simulink model "hil_sil_plant"  (R2022b)
settings: Solver=FixedStepAuto  StartTime=0.0  StopTime=inf  FixedStep=0.001  RelTol=1e-3
undefined symbols (not defined in the file): Ended, ind, Single
libraries: canmsglib x8, speedgoatlib_IO614 x5, speedgoatlib_IO191 x5, slrealtimeiplib x3, AMK_comms_plant_lib x1, BMS_plant_lib x1, slrealtimeutilitieslib x1, etargetslib x1
settings Model: Creator=LinF  LastModifiedBy=maxfa
settings SolverCC: ConcurrentTasks=on  PositivePriorityOrder=on
settings OptimizationCC: BlockReduction=off  OptimizeBlockIOStorage=off
settings DebuggingCC: TasksWithSamePriorityMsg=none
settings HardwareCC: ProdBitPerLong=64  ProdLongLongMode=on  ProdHWDeviceType=Intel->x86-64 (Linux 64)
settings RTWCC: Description=Simulink Real-Time  SystemTargetFile=slrealtime.tlc  TemplateMakefile=slrealtime_default_tmf  Toolchain=Simulink Real-Time Toolchain  BuildConfiguration=Faster Runs  CodeExecutionProfiling=on  TargetLang=C++

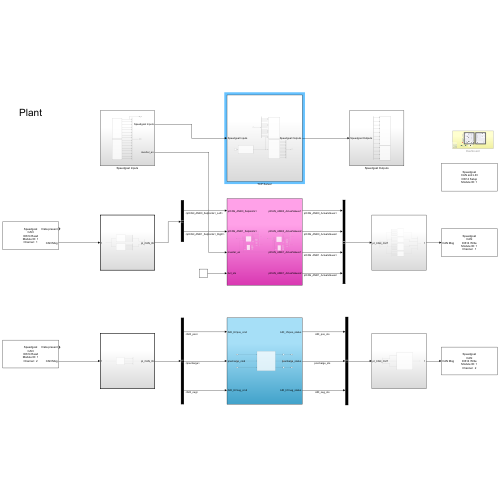
[thumbnail: Simulink's stored preview of the top-level diagram]
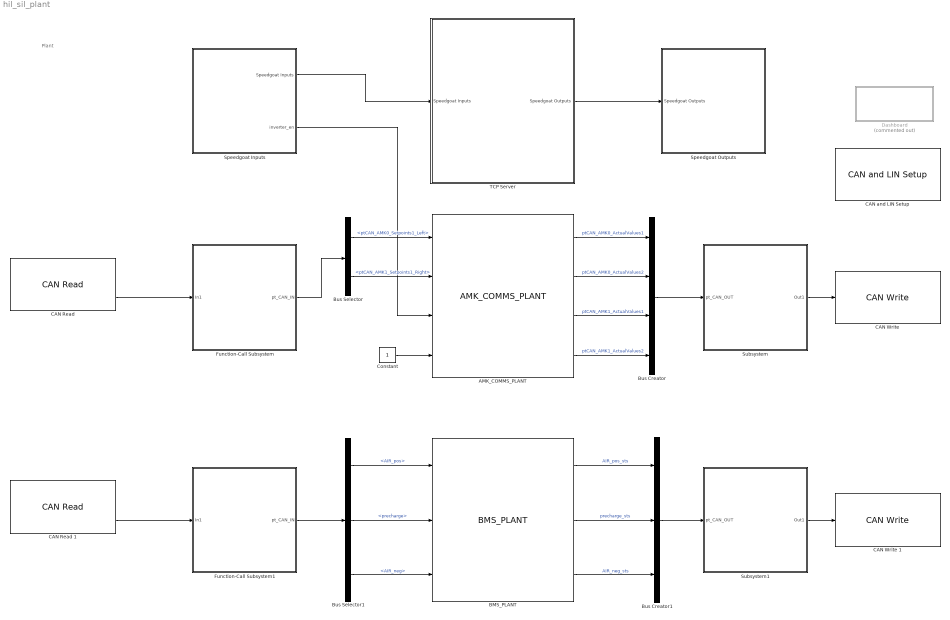
== system hil_sil_plant ==
  note: Plant
  AMK_COMMS_PLANT : AMK_comms_plant_lib/AMK_COMMS_PLANT  SystemSampleTime=-1  VariantActivationTime=update diagram  Latency=0  AutoFrameSizeCalculation=off
  BMS_PLANT : BMS_plant_lib/BMS_PLANT  SystemSampleTime=-1  VariantActivationTime=update diagram  Latency=0  AutoFrameSizeCalculation=off
  Bus Creator : BusCreator  Inputs=4
  Bus Creator1 : BusCreator  Inputs=3
  Bus Selector : BusSelector  OutputSignals=ptCAN_AMK0_Setpoints1_Left,ptCAN_AMK1_Setpoints1_Right
  Bus Selector1 : BusSelector  OutputSignals=AIR_pos,precharge,AIR_neg
  "CAN Read " : speedgoatlib_IO614/CAN Read   moduleType=IO614  id=1  channel=1  canType=CAN (HS)  useBusOut=off  HasMulRead=Single Read from Buffer (FIFO)  MsgIDlist=[1 2]  isEFF=off  LabelInHex=on  enableInput=off  ts=-1  initValues=[614 1 -1 0 1 1 0 0 0 1 2 1 2]
      settings: SourceProductName=Simulink Real-Time: Speedgoat I/O Blockset
  CAN Read 1 : speedgoatlib_IO614/CAN Read   moduleType=IO614  id=1  channel=2  canType=CAN (HS)  useBusOut=off  HasMulRead=Single Read from Buffer (FIFO)  MsgIDlist=[1 2]  isEFF=off  LabelInHex=on  enableInput=off  ts=-1  initValues=[614 1 -1 1 1 1 0 0 0 1 2 1 2]
      settings: SourceProductName=Simulink Real-Time: Speedgoat I/O Blockset
  "CAN Write " : speedgoatlib_IO614/CAN Write   moduleType=IO614  id=1  channel=1  canType=CAN (HS)  useBusIn=off  numOfMsg=4  enableInput=off  enableStatusPort=off  initValues=[614 1 0.01 0 1 1 0 4 0 0]  ts=0.01
      settings: SourceProductName=Simulink Real-Time: Speedgoat I/O Blockset
  CAN Write 1 : speedgoatlib_IO614/CAN Write   moduleType=IO614  id=1  channel=2  canType=CAN (HS)  useBusIn=off  numOfMsg=1  enableInput=off  enableStatusPort=off  initValues=[614 1 0.008 1 1 1 0 1 0 0]  ts=0.008
      settings: SourceProductName=Simulink Real-Time: Speedgoat I/O Blockset
  "CAN and LIN Setup " : speedgoatlib_IO614/CAN and LIN Setup   moduleInitValues="[614    1    1   -1   -1]"  id=1  moduleType=IO614  pciSlot=-1  canChn1=CAN (HS)  canChn2=CAN (HS)  canChn3=Disabled  canChn4=Disabled  linChn1=Disabled  linChn2=Disabled  canInitStructArray=[]  canTermStructArray=[]  canChn1InitValues="[2   4   1  31   8   2   1   5   2]"  arbBdrChn1=500 kBaud  arbManBdrChn1=[4,1,31,8]  fdBdrChn1=5.0 MBaud  fdManBdrChn1=[2,1,5,2]  canChn2InitValues="[2   4   1  31   8   2   1   5   2]"  arbBdrChn2=500 kBaud  arbManBdrChn2=[4,1,31,8]  fdBdrChn2=5.0 MBaud  fdManBdrChn2=[2,1,5,2]  canChn3InitValues="[1   2   1  31   8   2   1   5   2]"  arbBdrChn3=1.0 MBaud  arbManBdrChn3=[2,1,31,8]  fdBdrChn3=5.0 MBaud  fdManBdrChn3=[2,1,5,2]  canChn4InitValues="[1   2   1  31   8   2   1   5   2]"  arbBdrChn4=1.0 MBaud  arbManBdrChn4=[2,1,31,8]  fdBdrChn4=5.0 MBaud  fdManBdrChn4=[2,1,5,2]  bdrLIN1=19200  linChn1InitValues="[1  19200]"  bdrLIN2=19200  linChn2InitValues="[1  19200]"
      settings: LibrarySourceBlock=speedgoatlib_CANLIN_OfA2/CAN and LIN Setup
  Constant : Constant
  Dashboard : Subsystem  Commented=on
  Function-Call Subsystem : Subsystem  TreatAsAtomicUnit=on
  Function-Call Subsystem1 : Subsystem  TreatAsAtomicUnit=on
  Speedgoat Inputs : Subsystem
  Speedgoat Outputs : Subsystem
  Subsystem : Subsystem
  Subsystem1 : Subsystem
  TCP Server : Subsystem
  wires:
  Subsystem/1(Out1) -> "CAN Write "/1
  Function-Call Subsystem/1(pt_CAN_IN) -> Bus Selector/1
  Bus Selector/2 -> AMK_COMMS_PLANT/2  "<ptCAN_AMK1_Setpoints1_Right>"
  Bus Selector/1 -> AMK_COMMS_PLANT/1  "<ptCAN_AMK0_Setpoints1_Left>"
  Speedgoat Inputs/2(inverter_en) -> AMK_COMMS_PLANT/3
  AMK_COMMS_PLANT/1 -> Bus Creator/1  "ptCAN_AMK0_ActualValues1"
  AMK_COMMS_PLANT/2 -> Bus Creator/2  "ptCAN_AMK0_ActualValues2"
  AMK_COMMS_PLANT/3 -> Bus Creator/3  "ptCAN_AMK1_ActualValues1"
  AMK_COMMS_PLANT/4 -> Bus Creator/4  "ptCAN_AMK1_ActualValues2"
  Bus Creator/1 -> Subsystem/1(pt_CAN_OUT)
  Function-Call Subsystem1/1(pt_CAN_IN) -> Bus Selector1/1
  Bus Selector1/1 -> BMS_PLANT/1  "<AIR_pos>"
  Bus Selector1/3 -> BMS_PLANT/3  "<AIR_neg>"
  Subsystem1/1(Out1) -> CAN Write 1/1
  BMS_PLANT/1 -> Bus Creator1/1  "AIR_pos_sts"
  BMS_PLANT/2 -> Bus Creator1/2  "precharge_sts"
  BMS_PLANT/3 -> Bus Creator1/3  "AIR_neg_sts"
  Bus Creator1/1 -> Subsystem1/1(pt_CAN_OUT)
  "CAN Read "/2 -> Function-Call Subsystem/1(In1)
  CAN Read 1/2 -> Function-Call Subsystem1/1(In1)
  Bus Selector1/2 -> BMS_PLANT/2  "<precharge>"
  Constant/1 -> AMK_COMMS_PLANT/4
  TCP Server/1(Speedgoat Outputs) -> Speedgoat Outputs/1(Speedgoat Outputs)
  Speedgoat Inputs/1(Speedgoat Inputs) -> TCP Server/1(Speedgoat Inputs)

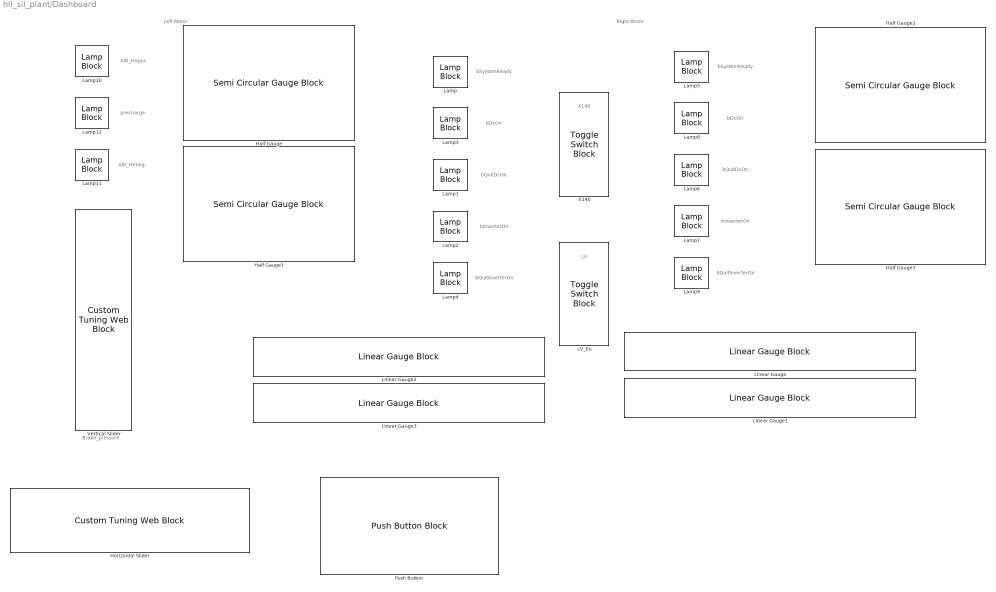
== system hil_sil_plant/Dashboard ==
  note: Brake_pressure
  note: LV
  note: X140
  note: Left Motor
  note: bQuitInverterOn
  note: bInverterOn
  note: bQuitDcOn
  note: bDcOn
  note: bSystemReady
  note: bDcOn
  note: bQuitDcOn
  note: bSystemReady
  note: bInverterOn
  note: bQuitInverterOn
  note: Right Motor
  note: AIR_HVpos
  note: precharge
  note: AIR_HVneg
  Half Gauge : SemiCircularGaugeBlock  LabelPosition=Bottom  ScaleMax=20000  TickInterval=2000
  Half Gauge1 : SemiCircularGaugeBlock  LabelPosition=Bottom  ScaleMax=1000  TickInterval=100
  Half Gauge2 : SemiCircularGaugeBlock  LabelPosition=Bottom  ScaleMax=20000  TickInterval=2000
  Half Gauge3 : SemiCircularGaugeBlock  LabelPosition=Bottom  ScaleMax=1000  TickInterval=100
  Horizontal Slider : CustomTuningWebBlock  LabelPosition=Hide  ShowInitialText=on  Configuration="{\"components\":[{\"name\":\"LinearScaleComponent\",\"settings\":{\"bounds\":{\"max\":4095,\"min\":0,\"tickInterval\":\"auto\"},\"internalTickHeightScaleFactor\":0.5,\"labelColor\":[255,255,200],\"labelFont\":{\"font\":\"Arial\",\"fontSize\":12},\"labelOffset\":0.05,\"labelTransparency\":1,\"needleImage\":{\"size\":[596,842],\"src\":\"data:image\\/svg+xml;base64,PD94bWwgdmVyc2lvbj0iMS4wIiBlbmNvZGluZz0idXRmLTgiPz4NCjwhLS0gR2VuZXJhdG9yOiBBZG9iZSBJbGx1c3RyYXRvciAyNS4wLjAsIFNWRyBFeHBvcnQgUGx1Zy1JbiAuIFNWRyBWZXJzaW9uOiA2LjAwIEJ1aWxkIDApICAtLT4NCjxzdmcgdmVyc2lvbj0iMS4xIg0KCSBpZD0ic3ZnOCIgeG1sbnM6Y2M9Imh0dHA6Ly9jcmVhdGl2ZWNvbW1vbnMub3JnL25zIyIgeG1sbnM6ZGM9Imh0dHA6Ly9wdXJsLm9yZy9kYy9lbGVtZW50cy8xLjEvIiB4bWxuczppbmtzY2FwZT0iaHR0cDovL3d3dy5pbmtzY2FwZS5vcmcvbmFtZXNw ...(+2420 chars)\",\"srcOrientation\":\"Right\"},\"needleOffset\":[-0.8044596912521441,-0.0642123287671233],\"needleSize\":{\"height\":0.4337797619047619,\"width\":0.07668067226890757},\"position\":[0.2829861111111111,0.04398634453781513,0.9196428571428571,0.6088789682539683],\"referencePoint\":\"auto\",\"scaleColors\":[],\"scaleColorsSize\":0.2,\"scaleDirection\":\"LR\",\"showLabels\":1,\"showMinorTicks\":0,\"showSpanLine\":1,\"showTicks\":1,\"tickColor\":[252,252,197],\"tickTransparency\":1,\"valueBarColor\":[0,114,189],\"valueBarOffset\":-0.27,\"valueBarSize\":0.1,\"valueBarTransparency\":1}},{\"name\":\"BackgroundImageComponent\",\"settings\":{\"image\":{\"size\":[380,101],\"src\":\"data:image\\/svg+xml;base64,PHN2ZyB4bWxucz0iaHR0cDovL3d3dy53My5vcmcvMjAwMC9zdmciIHhtbG5zOnhsaW5rPSJodHRwOi8vd3d3LnczLm9yZy8xOTk5L3hsaW5rIiB2aWV3Qm94PSIwIDAgMzgwIDEwMSI+PGRlZnM+PHN0eWxlPi5jbHMtMXtmaWxsOiMwMDJiNDI7fS5jbHMtMntmaWxsOiM0MjcwODI7fS5jbHMtM3tmaWxsOnVybCgjcmFkaWFsLWdyYWRpZW50KTt9LmNscy00e2ZpbGw6I2M4YzhjODtzdHJva2U6IzAwMDt9PC9zdHlsZT48cmFkaWFsR3JhZGllbnQgaWQ9InJhZGlhbC1ncmFkaWVudCIgY3g9IjE5MCIgY3k9IjUwLjUiIHI9IjI2OS4yMSIgZ3JhZGllbnRVbml0cz0idXNlclNwYWNlT25Vc2UiPjxzdG9wIG9mZnNldD0iMC4wMSIgc3RvcC1jb2xvcj0iIzNlNGY1OCIvPjxzdG9wIG9mZnNldD0iMC4wNiIgc3RvcC1jb2xvcj0iIzQ0NTc2MSIvPjxzdG9wIG9mZnNldD0iMC4xNSIgc3RvcC1jb2xvcj0iIzU1NmE3NiIvPjxzdG9wIG9mZnNldD0iMC4yNSIgc3RvcC1jb2xvcj0iIzZkODg5NSIvPjxzdG9wIG9mZnNldD0iMC4zOCIgc3RvcC1jb2xvcj0iIzhmYjJjMyIvPjxzdG9wIG9mZnNldD0iMC41MiIgc3RvcC1jb2xvcj0iI2I2ZTRmYSIvPjxzdG9wIG9mZnNldD0iMSIgc3RvcC1jb2xvcj0iIzE1NDY1NyIvPjwvcmFkaWFsR3JhZGllbnQ+PC9kZWZzPjxnIGlkPSJmcmFtZSI+PGcgaWQ9IkxheWVyXzIiIGRhdGEtbmFtZT0iTGF5ZXIgMiI+PGcgaWQ9IkxheWVyXzEtMiIgZGF0YS1uYW1lPSJMYXllciAxLTIiPjxyZWN0IGlkPSJyZWN0MTAzNiIgY2xhc3M9ImNscy0xIiB4PSIxMSIgeT0iMTEiIHdpZHRoPSIzNTgiIGhlaWdodD0iNzkiLz48cGF0aCBpZD0icGF0aDEwMzgiIGNsYXNzPSJjbHMtMiIgZD0iTTgsOFY5M0gzNzJWOFpNMzY5LDkwSDExVjExSDM2OVoiLz48cGF0aCBpZD0icGF0aDEwNDAiIGNsYXNzPSJjbHMtMyIgZD0iTTAsMFYxMDFIMzgwVjBaTTM3Miw5M0g4VjhIMzcyWiIvPjwvZz48L2c+PC9nPjxnIGlkPSJ0cmFjayI+PHBhdGggaWQ9InJlY3QxNjExIiBjbGFzcz0iY2xzLTQiIGQ9Ik0zMy4zNywyNi41OUgzNDYuNjNjNCwwLDcuMjUsMi42LDcuMjUsNS44MWgwYzAsMy4yMS0zLjI1LDUuODItNy4yNSw1LjgySDMzLjM3Yy00LDAtNy4yNS0yLjYxLTcuMjUtNS44MmgwQzI2LjEyLDI5LjE5LDI5LjM3LDI2LjU5LDMzLjM3LDI2LjU5WiIvPjwvZz48L3N2Zz4=\",\"srcOrientation\":\"horizontal\"},\"position\":[0,0,1,1],\"scaleMode\":\"0\"}},{\"name\":\"ForegroundImageComponent\",\"settings\":{\"image\":{\"size\":[0,0],\"src\":\"default\",\"srcOrientation\":[]},\"isForeground\":1,\"position\":[0,0,1,1],\"scaleMode\":\"0\"}}],\"settings\":{\"BindingType\":\"param\",\"aspectRatio\":3.7777777777777777,\"backgroundColor\":[0,0,0,\"1\"],\"backgroundOffset\":0,\"backgroundOpacity\":1,\"fixedAspectRatio\":\"on\",\"foregroundColor\":[252,252,196],\"orientation\":\"horizontal\",\"showBackgroundColor\":false,\"value\":0,\"version\":\"R2022b\"},\"type\":\"LinearGauge\"}"
  LV_En : ToggleSwitchBlock  LabelPosition=Bottom
      settings: Values={{'Off', 'On'}, [0 1]}
  Lamp{,1..12} (13 alike) : LampBlock  LabelPosition=Hide
  Linear Gauge : LinearGaugeBlock  ScaleMax=20000  TickInterval=2000
  Linear Gauge1 : LinearGaugeBlock  ScaleMax=1000  TickInterval=100
  Linear Gauge2 : LinearGaugeBlock  ScaleMax=20000  TickInterval=2000
  Linear Gauge3 : LinearGaugeBlock  ScaleMax=1000  TickInterval=100
  Push Button : PushButtonBlock  OffValue=-nan(ind)
  Vertical Slider : CustomTuningWebBlock  LabelPosition=Hide  ShowInitialText=on  Configuration="{\"components\":[{\"name\":\"LinearScaleComponent\",\"settings\":{\"bounds\":{\"max\":4095,\"min\":0,\"tickInterval\":\"auto\"},\"internalTickHeightScaleFactor\":0.5,\"labelColor\":[255,255,200],\"labelFont\":{\"font\":\"Arial\",\"fontSize\":12},\"labelOffset\":0.05,\"labelTransparency\":1,\"needleImage\":{\"size\":[596,842],\"src\":\"data:image\\/svg+xml;base64,PD94bWwgdmVyc2lvbj0iMS4wIiBlbmNvZGluZz0idXRmLTgiPz4NCjwhLS0gR2VuZXJhdG9yOiBBZG9iZSBJbGx1c3RyYXRvciAyNS4wLjAsIFNWRyBFeHBvcnQgUGx1Zy1JbiAuIFNWRyBWZXJzaW9uOiA2LjAwIEJ1aWxkIDApICAtLT4NCjxzdmcgdmVyc2lvbj0iMS4xIg0KCSBpZD0ic3ZnOCIgeG1sbnM6Y2M9Imh0dHA6Ly9jcmVhdGl2ZWNvbW1vbnMub3JnL25zIyIgeG1sbnM6ZGM9Imh0dHA6Ly9wdXJsLm9yZy9kYy9lbGVtZW50cy8xLjEvIiB4bWxuczppbmtzY2FwZT0iaHR0cDovL3d3dy5pbmtzY2FwZS5vcmcvbmFtZXNw ...(+2420 chars)\",\"srcOrientation\":\"horizontal\"},\"needleOffset\":[0.0642123287671233,-0.8044596912521441],\"needleSize\":{\"height\":0.07668067226890757,\"width\":0.4337797619047619},\"position\":[0.03623949579831933,0.2829861111111111,0.6088789682539683,0.9196428571428571],\"referencePoint\":\"auto\",\"scaleColors\":[],\"scaleColorsSize\":0.2,\"scaleDirection\":\"BT\",\"showLabels\":1,\"showMinorTicks\":0,\"showSpanLine\":1,\"showTicks\":1,\"tickColor\":[252,252,197],\"tickTransparency\":1,\"valueBarColor\":[0,114,189],\"valueBarOffset\":-0.27,\"valueBarSize\":0.1,\"valueBarTransparency\":1}},{\"name\":\"BackgroundImageComponent\",\"settings\":{\"image\":{\"size\":[380,101],\"src\":\"data:image\\/svg+xml;base64,PHN2ZyB4bWxucz0iaHR0cDovL3d3dy53My5vcmcvMjAwMC9zdmciIHhtbG5zOnhsaW5rPSJodHRwOi8vd3d3LnczLm9yZy8xOTk5L3hsaW5rIiB2aWV3Qm94PSIwIDAgMzgwIDEwMSI+PGRlZnM+PHN0eWxlPi5jbHMtMXtmaWxsOiMwMDJiNDI7fS5jbHMtMntmaWxsOiM0MjcwODI7fS5jbHMtM3tmaWxsOnVybCgjcmFkaWFsLWdyYWRpZW50KTt9LmNscy00e2ZpbGw6I2M4YzhjODtzdHJva2U6IzAwMDt9PC9zdHlsZT48cmFkaWFsR3JhZGllbnQgaWQ9InJhZGlhbC1ncmFkaWVudCIgY3g9IjE5MCIgY3k9IjUwLjUiIHI9IjI2OS4yMSIgZ3JhZGllbnRVbml0cz0idXNlclNwYWNlT25Vc2UiPjxzdG9wIG9mZnNldD0iMC4wMSIgc3RvcC1jb2xvcj0iIzNlNGY1OCIvPjxzdG9wIG9mZnNldD0iMC4wNiIgc3RvcC1jb2xvcj0iIzQ0NTc2MSIvPjxzdG9wIG9mZnNldD0iMC4xNSIgc3RvcC1jb2xvcj0iIzU1NmE3NiIvPjxzdG9wIG9mZnNldD0iMC4yNSIgc3RvcC1jb2xvcj0iIzZkODg5NSIvPjxzdG9wIG9mZnNldD0iMC4zOCIgc3RvcC1jb2xvcj0iIzhmYjJjMyIvPjxzdG9wIG9mZnNldD0iMC41MiIgc3RvcC1jb2xvcj0iI2I2ZTRmYSIvPjxzdG9wIG9mZnNldD0iMSIgc3RvcC1jb2xvcj0iIzE1NDY1NyIvPjwvcmFkaWFsR3JhZGllbnQ+PC9kZWZzPjxnIGlkPSJmcmFtZSI+PGcgaWQ9IkxheWVyXzIiIGRhdGEtbmFtZT0iTGF5ZXIgMiI+PGcgaWQ9IkxheWVyXzEtMiIgZGF0YS1uYW1lPSJMYXllciAxLTIiPjxyZWN0IGlkPSJyZWN0MTAzNiIgY2xhc3M9ImNscy0xIiB4PSIxMSIgeT0iMTEiIHdpZHRoPSIzNTgiIGhlaWdodD0iNzkiLz48cGF0aCBpZD0icGF0aDEwMzgiIGNsYXNzPSJjbHMtMiIgZD0iTTgsOFY5M0gzNzJWOFpNMzY5LDkwSDExVjExSDM2OVoiLz48cGF0aCBpZD0icGF0aDEwNDAiIGNsYXNzPSJjbHMtMyIgZD0iTTAsMFYxMDFIMzgwVjBaTTM3Miw5M0g4VjhIMzcyWiIvPjwvZz48L2c+PC9nPjxnIGlkPSJ0cmFjayI+PHBhdGggaWQ9InJlY3QxNjExIiBjbGFzcz0iY2xzLTQiIGQ9Ik0zMy4zNywyNi41OUgzNDYuNjNjNCwwLDcuMjUsMi42LDcuMjUsNS44MWgwYzAsMy4yMS0zLjI1LDUuODItNy4yNSw1LjgySDMzLjM3Yy00LDAtNy4yNS0yLjYxLTcuMjUtNS44MmgwQzI2LjEyLDI5LjE5LDI5LjM3LDI2LjU5LDMzLjM3LDI2LjU5WiIvPjwvZz48L3N2Zz4=\",\"srcOrientation\":\"horizontal\"},\"position\":[0,0,1,1],\"scaleMode\":\"0\"}},{\"name\":\"ForegroundImageComponent\",\"settings\":{\"image\":{\"size\":[0,0],\"src\":\"default\",\"srcOrientation\":[]},\"isForeground\":1,\"position\":[0,0,1,1],\"scaleMode\":\"0\"}}],\"settings\":{\"BindingType\":\"param\",\"aspectRatio\":3.7777777777777777,\"backgroundColor\":[0,0,0,\"1\"],\"backgroundOffset\":0,\"backgroundOpacity\":1,\"fixedAspectRatio\":\"on\",\"foregroundColor\":[252,252,196],\"orientation\":\"vertical\",\"showBackgroundColor\":false,\"value\":0,\"version\":\"R2022b\"},\"type\":\"LinearGauge\"}"
  X140 : ToggleSwitchBlock  LabelPosition=Bottom
      settings: Values={{'Off', 'On'}, [0 1]}

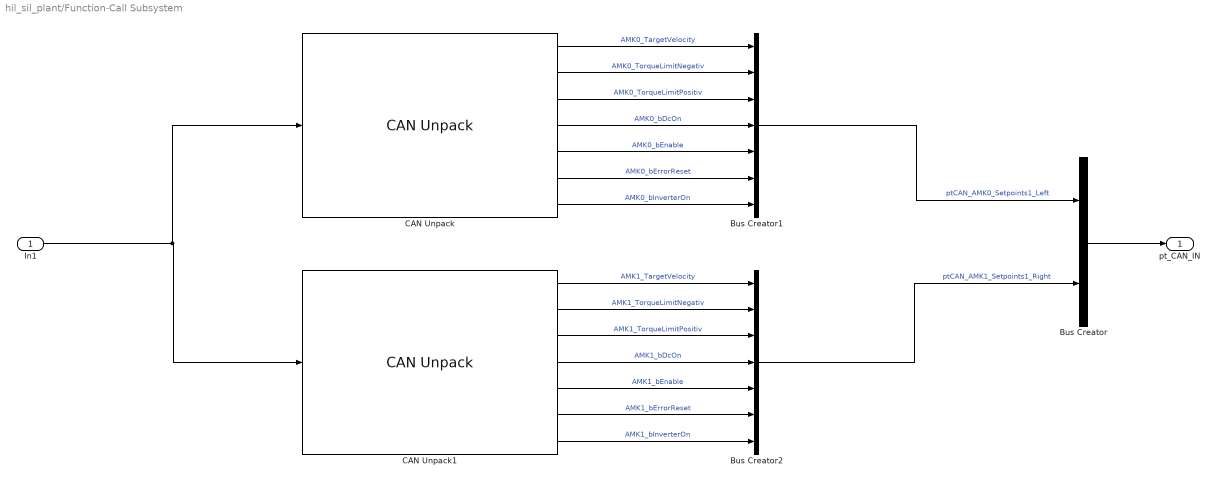
== system hil_sil_plant/Function-Call Subsystem ==
  In1 : Inport
  Bus Creator : BusCreator  Inputs=2
  Bus Creator1 : BusCreator  Inputs=7
  Bus Creator2 : BusCreator  Inputs=7
  CAN Unpack : canmsglib/CAN Unpack  CANdbFile=C:\Users\LinF\Documents\MACFE\Embedded\CAN_Stuff\CAN_Databases\CAN_AMKInverter.dbc  MsgList=(none)  MsgName=AMK0_SetPoints1  MsgIDType=Standard (11-bit identifier)  MsgIdentifier=389  MsgLength=8  SignalInfo={'AMK_TargetVelocity','16','16','LE','signed','Standard','0','1','0','-Inf','Inf';'AMK_TorqueLimitNegativ','48','16','LE','signed','Standard','0','1','0','-Inf','Inf';'AMK_TorqueLimitPositiv','32','16','LE','signed','Standard','0','1','0','-Inf','Inf';'AMK_bDcOn','9','1','LE','unsigned','Standard','0','1','0','-Inf','Inf';'AMK_bEnable','10','1','LE','unsigned','Standard','0','1','0','-Inf','Inf';'AMK_bErrorReset','11','1','LE','unsigned','Standard','0','1','0','-Inf','Inf';'AMK_bInverterOn','8','1','LE','unsigned','Standard','0','1','0','-Inf','Inf'}  IDPort=off  TimestampPort=off  ErrorPort=off  RemotePort=off  LengthPort=off  StatusPort=off  ApplyMinMax=off
      settings: LibrarySourceBlock=canlib/CAN Unpack  DataFormat=CANdb specified signals
  CAN Unpack1 : canmsglib/CAN Unpack  CANdbFile=C:\Users\LinF\Documents\MACFE\Embedded\CAN_Stuff\CAN_Databases\CAN_AMKInverter.dbc  MsgList=(none)  MsgName=AMK1_SetPoints1  MsgIDType=Standard (11-bit identifier)  MsgIdentifier=390  MsgLength=8  SignalInfo={'AMK_TargetVelocity','16','16','LE','signed','Standard','0','1','0','-Inf','Inf';'AMK_TorqueLimitNegativ','48','16','LE','signed','Standard','0','1','0','-Inf','Inf';'AMK_TorqueLimitPositiv','32','16','LE','signed','Standard','0','1','0','-Inf','Inf';'AMK_bDcOn','9','1','LE','unsigned','Standard','0','1','0','-Inf','Inf';'AMK_bEnable','10','1','LE','unsigned','Standard','0','1','0','-Inf','Inf';'AMK_bErrorReset','11','1','LE','unsigned','Standard','0','1','0','-Inf','Inf';'AMK_bInverterOn','8','1','LE','unsigned','Standard','0','1','0','-Inf','Inf'}  IDPort=off  TimestampPort=off  ErrorPort=off  RemotePort=off  LengthPort=off  StatusPort=off  ApplyMinMax=off
      settings: LibrarySourceBlock=canlib/CAN Unpack  DataFormat=CANdb specified signals
  pt_CAN_IN : Outport
  wires:
  Bus Creator/1 -> pt_CAN_IN/1
  Bus Creator2/1 -> Bus Creator/2  "ptCAN_AMK1_Setpoints1_Right"
  Bus Creator1/1 -> Bus Creator/1  "ptCAN_AMK0_Setpoints1_Left"
  In1/1 -> CAN Unpack/1, CAN Unpack1/1
  CAN Unpack/1 -> Bus Creator1/1  "AMK0_TargetVelocity"
  CAN Unpack/2 -> Bus Creator1/2  "AMK0_TorqueLimitNegativ"
  CAN Unpack/3 -> Bus Creator1/3  "AMK0_TorqueLimitPositiv"
  CAN Unpack/4 -> Bus Creator1/4  "AMK0_bDcOn"
  CAN Unpack/5 -> Bus Creator1/5  "AMK0_bEnable"
  CAN Unpack/6 -> Bus Creator1/6  "AMK0_bErrorReset"
  CAN Unpack/7 -> Bus Creator1/7  "AMK0_bInverterOn"
  CAN Unpack1/3 -> Bus Creator2/3  "AMK1_TorqueLimitPositiv"
  CAN Unpack1/6 -> Bus Creator2/6  "AMK1_bErrorReset"
  CAN Unpack1/4 -> Bus Creator2/4  "AMK1_bDcOn"
  CAN Unpack1/7 -> Bus Creator2/7  "AMK1_bInverterOn"
  CAN Unpack1/2 -> Bus Creator2/2  "AMK1_TorqueLimitNegativ"
  CAN Unpack1/5 -> Bus Creator2/5  "AMK1_bEnable"
  CAN Unpack1/1 -> Bus Creator2/1  "AMK1_TargetVelocity"

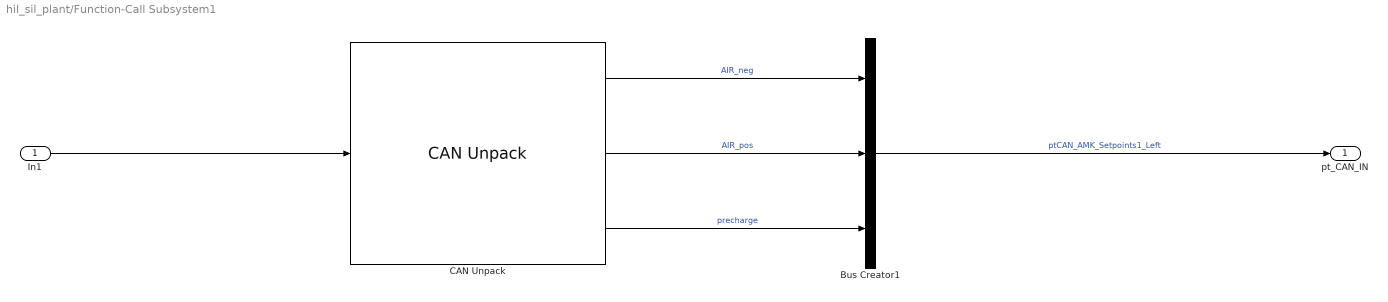
== system hil_sil_plant/Function-Call Subsystem1 ==
  In1 : Inport
  Bus Creator1 : BusCreator  Inputs=3
  CAN Unpack : canmsglib/CAN Unpack  CANdbFile=C:\Users\LinF\Documents\MACFE\Controls\repos\can_dbc\dbcs\VEH_CAN.dbc  MsgList=Contactor_States  MsgName=Contactor_States  MsgIDType=Standard (11-bit identifier)  MsgIdentifier=1570  MsgLength=3  SignalInfo={'Pack_Negative','16','8','LE','unsigned','Standard','0','1','0','-Inf','Inf';'Pack_Positive','0','8','LE','unsigned','Standard','0','1','0','-Inf','Inf';'Pack_Precharge','8','8','LE','unsigned','Standard','0','1','0','-Inf','Inf'}  IDPort=off  TimestampPort=off  ErrorPort=off  RemotePort=off  LengthPort=off  StatusPort=off  ApplyMinMax=off
      settings: LibrarySourceBlock=canlib/CAN Unpack  DataFormat=CANdb specified signals
  pt_CAN_IN : Outport
  wires:
  Bus Creator1/1 -> pt_CAN_IN/1  "ptCAN_AMK_Setpoints1_Left"
  In1/1 -> CAN Unpack/1
  CAN Unpack/3 -> Bus Creator1/3  "precharge"
  CAN Unpack/1 -> Bus Creator1/1  "AIR_neg"
  CAN Unpack/2 -> Bus Creator1/2  "AIR_pos"

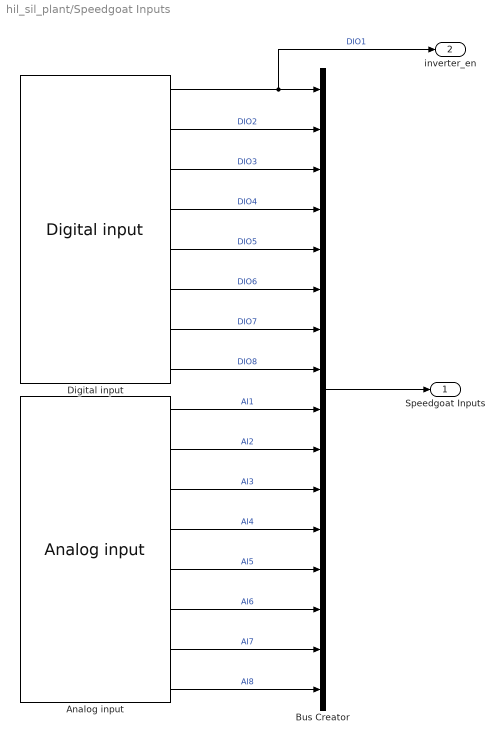
== system hil_sil_plant/Speedgoat Inputs ==
  "Analog input " : speedgoatlib_IO191/Analog input   parModuleId=1  parSampleTime=-1  parPciSlot=-1  parAdcChannels=[1 2 3 4 5 6 7 8]  parAdcMode=2  parAdcRanges=[4 4 4 4 4 4 4 4]  parAdcInitValues=[0 0]  parAdcResets=[1 1]  paramsAdcDma=[0 1 200 -1]
      settings: SourceProductName=Simulink Real-Time: Speedgoat I/O Blockset
  Bus Creator : BusCreator  Inputs=16
  "Digital input " : speedgoatlib_IO191/Digital input   parModuleId=1  parSampleTime=-1  parPciSlot=-1  parDiChannels=[1 2 3 4 5 6 7 8]
      settings: SourceProductName=Simulink Real-Time: Speedgoat I/O Blockset
  Speedgoat Inputs : Outport
  inverter_en : Outport  Port=2
  wires:
  Bus Creator/1 -> Speedgoat Inputs/1
  "Digital input "/1 -> inverter_en/1, Bus Creator/1  "DIO1"
  "Digital input "/2 -> Bus Creator/2  "DIO2"
  "Digital input "/3 -> Bus Creator/3  "DIO3"
  "Digital input "/4 -> Bus Creator/4  "DIO4"
  "Digital input "/5 -> Bus Creator/5  "DIO5"
  "Digital input "/6 -> Bus Creator/6  "DIO6"
  "Digital input "/7 -> Bus Creator/7  "DIO7"
  "Digital input "/8 -> Bus Creator/8  "DIO8"
  "Analog input "/1 -> Bus Creator/9  "AI1"
  "Analog input "/2 -> Bus Creator/10  "AI2"
  "Analog input "/3 -> Bus Creator/11  "AI3"
  "Analog input "/4 -> Bus Creator/12  "AI4"
  "Analog input "/5 -> Bus Creator/13  "AI5"
  "Analog input "/6 -> Bus Creator/14  "AI6"
  "Analog input "/7 -> Bus Creator/15  "AI7"
  "Analog input "/8 -> Bus Creator/16  "AI8"

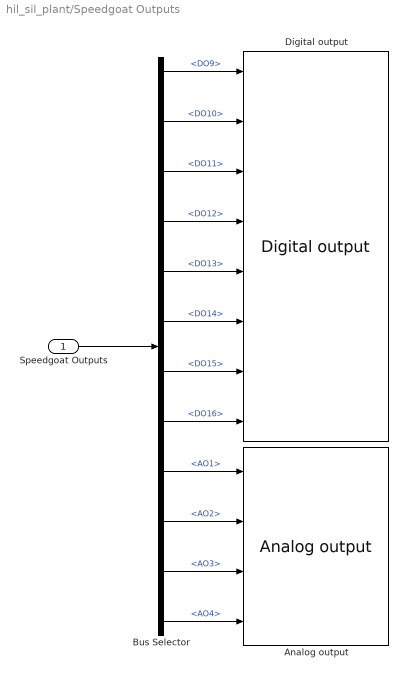
== system hil_sil_plant/Speedgoat Outputs ==
  Speedgoat Outputs : Inport
  "Analog output " : speedgoatlib_IO191/Analog output   parModuleId=1  parSampleTime=-1  parPciSlot=-1  parDacChannels=[1 2 3 4]  parModuleType=1  parDacRanges=[3 3 3 3]  parDacInitValues=[0 0 0 0]  parDacResets=[1 1 1 1]
      settings: SourceProductName=Simulink Real-Time: Speedgoat I/O Blockset
  Bus Selector : BusSelector  OutputSignals=DO9,DO10,DO11,DO12,DO13,DO14,DO15,DO16,AO1,AO2,AO3,AO4
  "Digital output " : speedgoatlib_IO191/Digital output   parModuleId=1  parSampleTime=-1  parPciSlot=-1  parDoChannels=[9 10 11 12 13 14 15 16]  parDoInitValues=[0 0 0 0 0 0 0 0]  parDoResets=[1 1 1 1 1 1 1 1]
      settings: SourceProductName=Simulink Real-Time: Speedgoat I/O Blockset
  wires:
  Speedgoat Outputs/1 -> Bus Selector/1
  Bus Selector/4 -> "Digital output "/4  "<DO12>"
  Bus Selector/1 -> "Digital output "/1  "<DO9>"
  Bus Selector/2 -> "Digital output "/2  "<DO10>"
  Bus Selector/5 -> "Digital output "/5  "<DO13>"
  Bus Selector/3 -> "Digital output "/3  "<DO11>"
  Bus Selector/6 -> "Digital output "/6  "<DO14>"
  Bus Selector/7 -> "Digital output "/7  "<DO15>"
  Bus Selector/8 -> "Digital output "/8  "<DO16>"
  Bus Selector/9 -> "Analog output "/1  "<AO1>"
  Bus Selector/10 -> "Analog output "/2  "<AO2>"
  Bus Selector/11 -> "Analog output "/3  "<AO3>"
  Bus Selector/12 -> "Analog output "/4  "<AO4>"

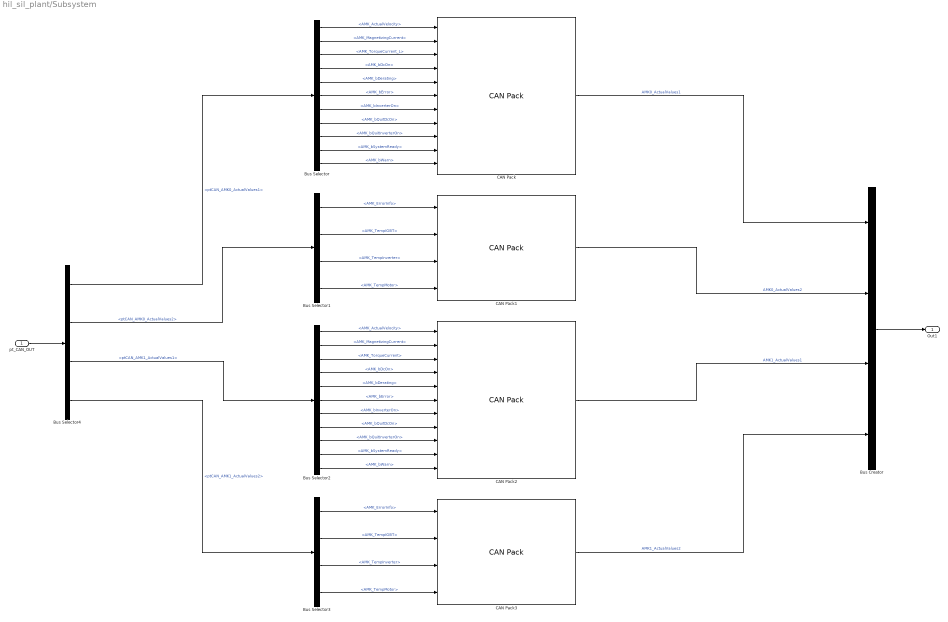
== system hil_sil_plant/Subsystem ==
  pt_CAN_OUT : Inport
  Bus Creator : BusCreator  Inputs=4
  Bus Selector : BusSelector  OutputSignals=AMK_ActualVelocity,AMK_MagnetizingCurrent,AMK_TorqueCurrent_L,AMK_bDcOn,AMK_bDerating,AMK_bError,AMK_bInverterOn,AMK_bQuitDcOn,AMK_bQuitInverterOn,AMK_bSystemReady,AMK_bWarn
  Bus Selector1 : BusSelector  OutputSignals=AMK_ErrorInfo,AMK_TempIGBT,AMK_TempInverter,AMK_TempMotor
  Bus Selector2 : BusSelector  OutputSignals=AMK_ActualVelocity,AMK_MagnetizingCurrent,AMK_TorqueCurrent,AMK_bDcOn,AMK_bDerating,AMK_bError,AMK_bInverterOn,AMK_bQuitDcOn,AMK_bQuitInverterOn,AMK_bSystemReady,AMK_bWarn
  Bus Selector3 : BusSelector  OutputSignals=AMK_ErrorInfo,AMK_TempIGBT,AMK_TempInverter,AMK_TempMotor
  Bus Selector4 : BusSelector  OutputSignals=ptCAN_AMK0_ActualValues1,ptCAN_AMK0_ActualValues2,ptCAN_AMK1_ActualValues1,ptCAN_AMK1_ActualValues2
  CAN Pack : canmsglib/CAN Pack  CANdbFile=C:\Users\LinF\Documents\MACFE\Embedded\CAN_Stuff\CAN_Databases\CAN_AMKInverter.dbc  MsgList=(none)  MsgName=AMK0_ActualValues1  MsgIDType=Standard (11-bit identifier)  MsgIdentifier=644  MsgLength=8  Remote=off  ApplyMinMax=off  BusOutput=off  SignalInfo={'AMK_ActualVelocity','16','16','LE','signed','Standard','0','1','0','-Inf','Inf';'AMK_MagnetizingCurrent','48','16','LE','signed','Standard','0','1','0','-Inf','Inf';'AMK_TorqueCurrent','32','16','LE','signed','Standard','0','1','0','-Inf','Inf';'AMK_bDcOn','12','1','LE','unsigned','Standard','0','1','0','-Inf','Inf';'AMK_bDerating','15','1','LE','unsigned','Standard','0','1','0','-Inf','Inf';'AMK_bError','9','1','LE','unsigned','Standard','0','1','0','-Inf','Inf';'AMK_bInverterOn','14','1','LE','unsigned','Standard','0','1','0','-Inf','Inf';'AMK_bQuitDcOn','11','1','LE','unsigned','Standard','0','1','0','-Inf','Inf';'AMK_bQuitInverterOn','13','1','LE','unsigned','Standard','0','1','0','-Inf','Inf';'AMK_bSystemReady','8','1','LE','unsigned','Standard','0','1','0','-Inf','Inf';'AMK_bWarn','10','1','LE','unsigned','Standard','0','1','0','-Inf','Inf'}
      settings: LibrarySourceBlock=canlib/CAN Pack  DataFormat=CANdb specified signals
  CAN Pack1 : canmsglib/CAN Pack  CANdbFile=C:\Users\LinF\Documents\MACFE\Embedded\CAN_Stuff\CAN_Databases\CAN_AMKInverter.dbc  MsgList=(none)  MsgName=AMK0_ActualValues2  MsgIDType=Standard (11-bit identifier)  MsgIdentifier=646  MsgLength=8  Remote=off  ApplyMinMax=off  BusOutput=off  SignalInfo={'AMK_ErrorInfo','32','16','LE','unsigned','Standard','0','1','0','0','65535';'AMK_TempIGBT','48','16','LE','signed','Standard','0','0.1','0','-3276.8','3276.7';'AMK_TempInverter','16','16','LE','signed','Standard','0','0.1','0','-3276.8','3276.7';'AMK_TempMotor','0','16','LE','signed','Standard','0','0.1','0','-3276.8','3276.7'}
      settings: LibrarySourceBlock=canlib/CAN Pack  DataFormat=CANdb specified signals
  CAN Pack2 : canmsglib/CAN Pack  CANdbFile=C:\Users\LinF\Documents\MACFE\Embedded\CAN_Stuff\CAN_Databases\CAN_AMKInverter.dbc  MsgList=(none)  MsgName=AMK1_ActualValues1  MsgIDType=Standard (11-bit identifier)  MsgIdentifier=645  MsgLength=8  Remote=off  ApplyMinMax=off  BusOutput=off  SignalInfo={'AMK_ActualVelocity','16','16','LE','signed','Standard','0','1','0','-Inf','Inf';'AMK_MagnetizingCurrent','48','16','LE','signed','Standard','0','1','0','-Inf','Inf';'AMK_TorqueCurrent','32','16','LE','signed','Standard','0','1','0','-Inf','Inf';'AMK_bDcOn','12','1','LE','unsigned','Standard','0','1','0','-Inf','Inf';'AMK_bDerating','15','1','LE','unsigned','Standard','0','1','0','-Inf','Inf';'AMK_bError','9','1','LE','unsigned','Standard','0','1','0','-Inf','Inf';'AMK_bInverterOn','14','1','LE','unsigned','Standard','0','1','0','-Inf','Inf';'AMK_bQuitDcOn','11','1','LE','unsigned','Standard','0','1','0','-Inf','Inf';'AMK_bQuitInverterOn','13','1','LE','unsigned','Standard','0','1','0','-Inf','Inf';'AMK_bSystemReady','8','1','LE','unsigned','Standard','0','1','0','-Inf','Inf';'AMK_bWarn','10','1','LE','unsigned','Standard','0','1','0','-Inf','Inf'}
      settings: LibrarySourceBlock=canlib/CAN Pack  DataFormat=CANdb specified signals
  CAN Pack3 : canmsglib/CAN Pack  CANdbFile=C:\Users\LinF\Documents\MACFE\Embedded\CAN_Stuff\CAN_Databases\CAN_AMKInverter.dbc  MsgList=(none)  MsgName=AMK1_ActualValues2  MsgIDType=Standard (11-bit identifier)  MsgIdentifier=647  MsgLength=8  Remote=off  ApplyMinMax=off  BusOutput=off  SignalInfo={'AMK_ErrorInfo','32','16','LE','unsigned','Standard','0','1','0','0','65535';'AMK_TempIGBT','48','16','LE','signed','Standard','0','0.1','0','-3276.8','3276.7';'AMK_TempInverter','16','16','LE','signed','Standard','0','0.1','0','-3276.8','3276.7';'AMK_TempMotor','0','16','LE','signed','Standard','0','0.1','0','-3276.8','3276.7'}
      settings: LibrarySourceBlock=canlib/CAN Pack  DataFormat=CANdb specified signals
  Out1 : Outport
  wires:
  CAN Pack/1 -> Bus Creator/1  "AMK0_ActualValues1"
  CAN Pack1/1 -> Bus Creator/2  "AMK0_ActualValues2"
  CAN Pack2/1 -> Bus Creator/3  "AMK1_ActualValues1"
  CAN Pack3/1 -> Bus Creator/4  "AMK1_ActualValues2"
  Bus Selector4/1 -> Bus Selector/1  "<ptCAN_AMK0_ActualValues1>"
  Bus Selector4/2 -> Bus Selector1/1  "<ptCAN_AMK0_ActualValues2>"
  Bus Selector4/3 -> Bus Selector2/1  "<ptCAN_AMK1_ActualValues1>"
  Bus Selector4/4 -> Bus Selector3/1  "<ptCAN_AMK1_ActualValues2>"
  pt_CAN_OUT/1 -> Bus Selector4/1
  Bus Creator/1 -> Out1/1
  Bus Selector/1 -> CAN Pack/1  "<AMK_ActualVelocity>"
  Bus Selector/3 -> CAN Pack/3  "<AMK_TorqueCurrent_L>"
  Bus Selector/2 -> CAN Pack/2  "<AMK_MagnetizingCurrent>"
  Bus Selector/4 -> CAN Pack/4  "<AMK_bDcOn>"
  Bus Selector/5 -> CAN Pack/5  "<AMK_bDerating>"
  Bus Selector/6 -> CAN Pack/6  "<AMK_bError>"
  Bus Selector/7 -> CAN Pack/7  "<AMK_bInverterOn>"
  Bus Selector/8 -> CAN Pack/8  "<AMK_bQuitDcOn>"
  Bus Selector/9 -> CAN Pack/9  "<AMK_bQuitInverterOn>"
  Bus Selector/10 -> CAN Pack/10  "<AMK_bSystemReady>"
  Bus Selector/11 -> CAN Pack/11  "<AMK_bWarn>"
  Bus Selector1/1 -> CAN Pack1/1  "<AMK_ErrorInfo>"
  Bus Selector1/2 -> CAN Pack1/2  "<AMK_TempIGBT>"
  Bus Selector1/3 -> CAN Pack1/3  "<AMK_TempInverter>"
  Bus Selector1/4 -> CAN Pack1/4  "<AMK_TempMotor>"
  Bus Selector2/3 -> CAN Pack2/3  "<AMK_TorqueCurrent>"
  Bus Selector3/1 -> CAN Pack3/1  "<AMK_ErrorInfo>"
  Bus Selector2/7 -> CAN Pack2/7  "<AMK_bInverterOn>"
  Bus Selector2/4 -> CAN Pack2/4  "<AMK_bDcOn>"
  Bus Selector2/2 -> CAN Pack2/2  "<AMK_MagnetizingCurrent>"
  Bus Selector3/4 -> CAN Pack3/4  "<AMK_TempMotor>"
  Bus Selector3/2 -> CAN Pack3/2  "<AMK_TempIGBT>"
  Bus Selector2/5 -> CAN Pack2/5  "<AMK_bDerating>"
  Bus Selector2/10 -> CAN Pack2/10  "<AMK_bSystemReady>"
  Bus Selector3/3 -> CAN Pack3/3  "<AMK_TempInverter>"
  Bus Selector2/8 -> CAN Pack2/8  "<AMK_bQuitDcOn>"
  Bus Selector2/6 -> CAN Pack2/6  "<AMK_bError>"
  Bus Selector2/11 -> CAN Pack2/11  "<AMK_bWarn>"
  Bus Selector2/1 -> CAN Pack2/1  "<AMK_ActualVelocity>"
  Bus Selector2/9 -> CAN Pack2/9  "<AMK_bQuitInverterOn>"

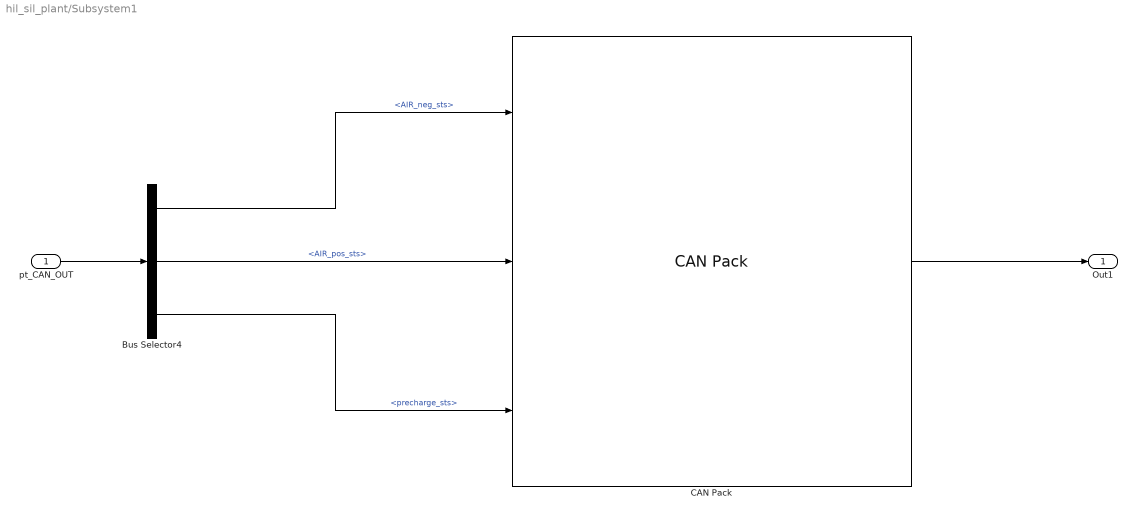
== system hil_sil_plant/Subsystem1 ==
  pt_CAN_OUT : Inport
  Bus Selector4 : BusSelector  OutputSignals=AIR_neg_sts,AIR_pos_sts,precharge_sts
  CAN Pack : canmsglib/CAN Pack  CANdbFile=C:\Users\LinF\Documents\MACFE\Controls\repos\can_dbc\dbcs\VEH_CAN.dbc  MsgList=Contactor_Feedback  MsgName=Contactor_Feedback  MsgIDType=Standard (11-bit identifier)  MsgIdentifier=1574  MsgLength=3  Remote=off  ApplyMinMax=off  BusOutput=off  SignalInfo={'Pack_Negative_Feedback','8','1','LE','unsigned','Standard','0','1','0','0','1';'Pack_Positive_Feedback','0','1','LE','unsigned','Standard','0','1','0','0','1';'Pack_Precharge_Feedback','16','1','LE','unsigned','Standard','0','1','0','0','1'}
      settings: LibrarySourceBlock=canlib/CAN Pack  DataFormat=CANdb specified signals
  Out1 : Outport
  wires:
  pt_CAN_OUT/1 -> Bus Selector4/1
  Bus Selector4/2 -> CAN Pack/2  "<AIR_pos_sts>"
  Bus Selector4/3 -> CAN Pack/3  "<precharge_sts>"
  Bus Selector4/1 -> CAN Pack/1  "<AIR_neg_sts>"
  CAN Pack/1 -> Out1/1

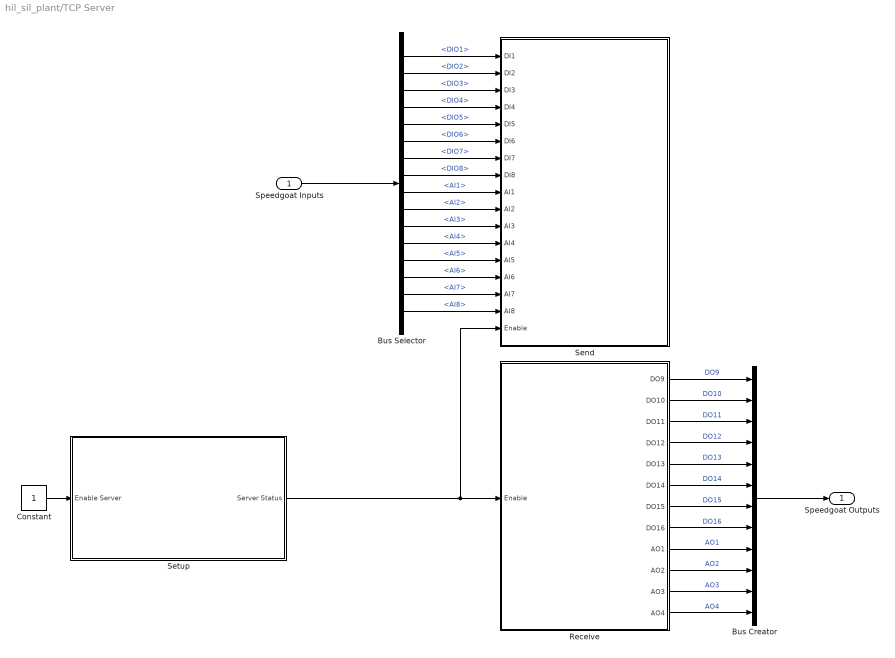
== system hil_sil_plant/TCP Server ==
  Speedgoat Inputs : Inport
  Bus Creator : BusCreator  Inputs=12
  Bus Selector : BusSelector  OutputSignals=DIO1,DIO2,DIO3,DIO4,DIO5,DIO6,DIO7,DIO8,AI1,AI2,AI3,AI4,AI5,AI6,AI7,AI8
  Constant : Constant
  Receive : Subsystem
  Send : Subsystem
  Setup : Subsystem
  Speedgoat Outputs : Outport
  wires:
  Constant/1 -> Setup/1(Enable Server)
  Setup/1(Server Status) -> Send/17(Enable), Receive/1(Enable)
  Receive/1(DO9) -> Bus Creator/1  "DO9"
  Receive/2(DO10) -> Bus Creator/2  "DO10"
  Receive/3(DO11) -> Bus Creator/3  "DO11"
  Receive/4(DO12) -> Bus Creator/4  "DO12"
  Receive/5(DO13) -> Bus Creator/5  "DO13"
  Receive/6(DO14) -> Bus Creator/6  "DO14"
  Receive/7(DO15) -> Bus Creator/7  "DO15"
  Receive/8(DO16) -> Bus Creator/8  "DO16"
  Receive/9(AO1) -> Bus Creator/9  "AO1"
  Receive/10(AO2) -> Bus Creator/10  "AO2"
  Receive/11(AO3) -> Bus Creator/11  "AO3"
  Receive/12(AO4) -> Bus Creator/12  "AO4"
  Bus Creator/1 -> Speedgoat Outputs/1
  Speedgoat Inputs/1 -> Bus Selector/1
  Bus Selector/1 -> Send/1(DI1)  "<DIO1>"
  Bus Selector/2 -> Send/2(DI2)  "<DIO2>"
  Bus Selector/3 -> Send/3(DI3)  "<DIO3>"
  Bus Selector/4 -> Send/4(DI4)  "<DIO4>"
  Bus Selector/5 -> Send/5(DI5)  "<DIO5>"
  Bus Selector/6 -> Send/6(DI6)  "<DIO6>"
  Bus Selector/7 -> Send/7(DI7)  "<DIO7>"
  Bus Selector/8 -> Send/8(DI8)  "<DIO8>"
  Bus Selector/9 -> Send/9(AI1)  "<AI1>"
  Bus Selector/10 -> Send/10(AI2)  "<AI2>"
  Bus Selector/11 -> Send/11(AI3)  "<AI3>"
  Bus Selector/12 -> Send/12(AI4)  "<AI4>"
  Bus Selector/13 -> Send/13(AI5)  "<AI5>"
  Bus Selector/14 -> Send/14(AI6)  "<AI6>"
  Bus Selector/15 -> Send/15(AI7)  "<AI7>"
  Bus Selector/16 -> Send/16(AI8)  "<AI8>"

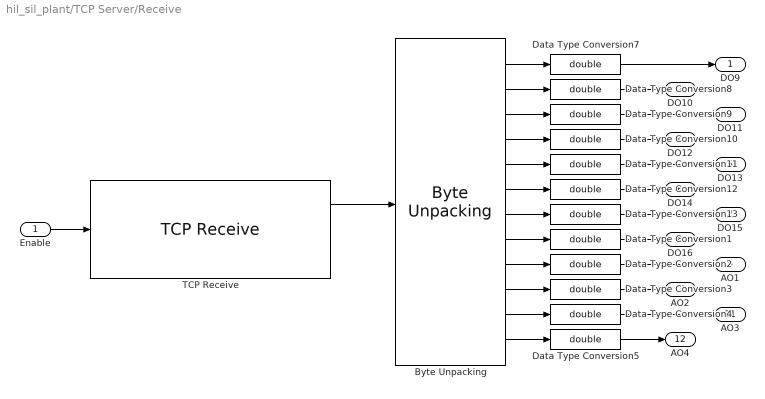
== system hil_sil_plant/TCP Server/Receive ==
  Enable : Inport
  Byte Unpacking : slrealtimeutilitieslib/Byte Unpacking  MaskUnpackedDataTypes={'uint8','uint8','uint8','uint8','uint8','uint8','uint8','uint8','double','double','double','double'}  MaskUnpackedDataSizes={1,1,1,1,1,1,1,1,1,1,1,1}  MaskAlignment=1
  Data Type Conversion{1..5,7..13} (12 alike) : DataTypeConversion  OutDataTypeStr=double  SaturateOnIntegerOverflow=off  RndMeth=Floor
  TCP Receive : slrealtimeiplib/TCP Receive  socketAddPortVal=Server: 192.168.10.1:8001  rcvWidth=40  sampleTime=0.01
  DO9 : Outport
  DO10 : Outport  Port=2
  DO11 : Outport  Port=3
  DO12 : Outport  Port=4
  DO13 : Outport  Port=5
  DO14 : Outport  Port=6
  DO15 : Outport  Port=7
  DO16 : Outport  Port=8
  AO1 : Outport  Port=9
  AO2 : Outport  Port=10
  AO3 : Outport  Port=11
  AO4 : Outport  Port=12
  wires:
  Enable/1 -> TCP Receive/1
  TCP Receive/1 -> Byte Unpacking/1
  Byte Unpacking/8 -> Data Type Conversion1/1
  Byte Unpacking/7 -> Data Type Conversion13/1
  Byte Unpacking/2 -> Data Type Conversion8/1
  Byte Unpacking/6 -> Data Type Conversion12/1
  Data Type Conversion8/1 -> DO10/1
  Data Type Conversion10/1 -> DO12/1
  Data Type Conversion9/1 -> DO11/1
  Byte Unpacking/5 -> Data Type Conversion11/1
  Byte Unpacking/1 -> Data Type Conversion7/1
  Byte Unpacking/3 -> Data Type Conversion9/1
  Data Type Conversion12/1 -> DO14/1
  Byte Unpacking/10 -> Data Type Conversion3/1
  Byte Unpacking/9 -> Data Type Conversion2/1
  Byte Unpacking/4 -> Data Type Conversion10/1
  Data Type Conversion13/1 -> DO15/1
  Data Type Conversion11/1 -> DO13/1
  Byte Unpacking/12 -> Data Type Conversion5/1
  Data Type Conversion7/1 -> DO9/1
  Byte Unpacking/11 -> Data Type Conversion4/1
  Data Type Conversion1/1 -> DO16/1
  Data Type Conversion2/1 -> AO1/1
  Data Type Conversion3/1 -> AO2/1
  Data Type Conversion4/1 -> AO3/1
  Data Type Conversion5/1 -> AO4/1

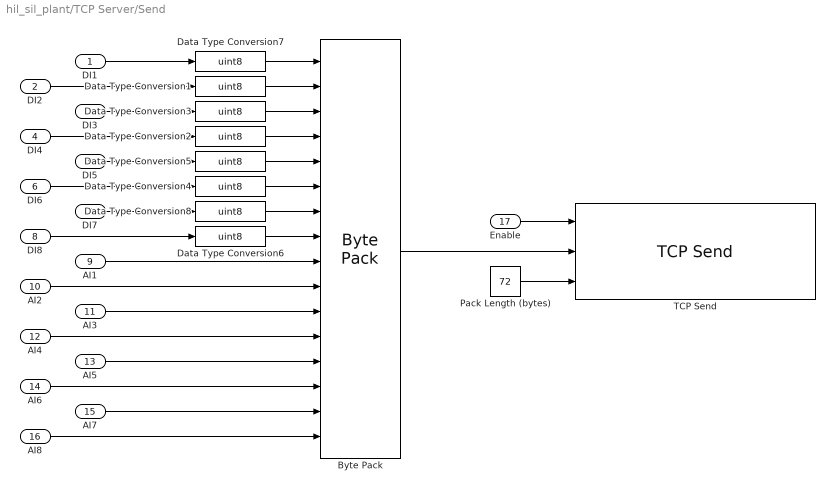
== system hil_sil_plant/TCP Server/Send ==
  DI1 : Inport
  DI2 : Inport  Port=2
  DI3 : Inport  Port=3
  DI4 : Inport  Port=4
  DI5 : Inport  Port=5
  DI6 : Inport  Port=6
  DI7 : Inport  Port=7
  DI8 : Inport  Port=8
  AI1 : Inport  Port=9
  AI2 : Inport  Port=10
  AI3 : Inport  Port=11
  AI4 : Inport  Port=12
  AI5 : Inport  Port=13
  AI6 : Inport  Port=14
  AI7 : Inport  Port=15
  AI8 : Inport  Port=16
  Enable : Inport  Port=17
  Byte Pack : etargetslib/Byte Pack  datatypes={'uint8','uint8','uint8','uint8','uint8','uint8','uint8','uint8','double','double','double','double','double','double','double','double'}  byteAlign=1
  Data Type Conversion{1..8} (8 alike) : DataTypeConversion  OutDataTypeStr=uint8  SaturateOnIntegerOverflow=off  RndMeth=Floor
  Pack Length (bytes) : Constant  Value=72
  TCP Send : slrealtimeiplib/TCP Send  socketAddPortVal=Server: 192.168.10.1:8001  sampleTime=0.01
  wires:
  Enable/1 -> TCP Send/1
  DI1/1 -> Data Type Conversion7/1
  DI2/1 -> Data Type Conversion1/1
  DI3/1 -> Data Type Conversion3/1
  DI4/1 -> Data Type Conversion2/1
  DI5/1 -> Data Type Conversion5/1
  DI6/1 -> Data Type Conversion4/1
  DI7/1 -> Data Type Conversion8/1
  DI8/1 -> Data Type Conversion6/1
  AI1/1 -> Byte Pack/9
  AI2/1 -> Byte Pack/10
  AI3/1 -> Byte Pack/11
  AI4/1 -> Byte Pack/12
  Byte Pack/1 -> TCP Send/2
  Data Type Conversion7/1 -> Byte Pack/1
  Data Type Conversion1/1 -> Byte Pack/2
  Data Type Conversion3/1 -> Byte Pack/3
  Data Type Conversion2/1 -> Byte Pack/4
  Data Type Conversion4/1 -> Byte Pack/6
  Data Type Conversion5/1 -> Byte Pack/5
  Data Type Conversion6/1 -> Byte Pack/8
  Data Type Conversion8/1 -> Byte Pack/7
  AI5/1 -> Byte Pack/13
  AI6/1 -> Byte Pack/14
  AI7/1 -> Byte Pack/15
  AI8/1 -> Byte Pack/16
  Pack Length (bytes)/1 -> TCP Send/3

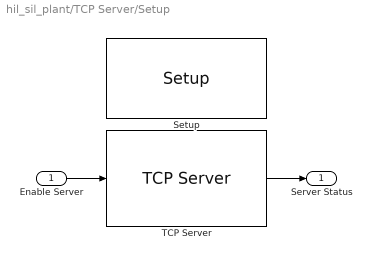
== system hil_sil_plant/TCP Server/Setup ==
  Enable Server : Inport
  "Setup " : speedgoatlib_IO191/Setup   parModuleId=1  parPciSlot=-1  parTriggerSignal=TTL  parAdcChannels=[1 2 3 4 5 6 7 8]  parAdcRanges=[4 4 4 4 4 4 4 4]  parAdcChannel1=on  parAdcChannel2=on  parAdcChannel3=on  parAdcChannel4=on  parAdcChannel5=on  parAdcChannel6=on  parAdcChannel7=on  parAdcChannel8=on  parAdcMode=Single-Ended  parAdcRange11=+-5.12 V  parAdcRange21=+-24.576 V  parAdcRange12=+-5.12 V  parAdcRange22=+-24.576 V  parAdcRange13=+-5.12 V  parAdcRange23=+-24.576 V  parAdcRange14=+-5.12 V  parAdcRange24=+-24.576 V  parAdcRange15=+-5.12 V  parAdcRange25=+-24.576 V  parAdcRange16=+-5.12 V  parAdcRange26=+-24.576 V  parAdcRange17=+-5.12 V  parAdcRange27=+-24.576 V  parAdcRange18=+-5.12 V  parAdcRange28=+-24.576 V  parAdcEnDma=off  parAdcFrame=125  parAdcDiv=200  parAdcSample=-1  parDacChannels=[1 2 3 4]  parDacChannel1=on  parDacChannel2=on  parDacChannel3=on  parDacChannel4=on  parDacMode=Single-Ended  parDacRanges=[3 3 3 3]  parDacInitValues=[0 0 0 0]  parDacResets=[1 1 1 1]  parDacRange1=+-5 V  parDacInitValue1=0  parDacReset1=on  parDacRange2=+-5 V  parDacInitValue2=0  parDacReset2=on  parDacRange3=+-5 V  parDacInitValue3=0  parDacReset3=on  parDacRange4=+-5 V  parDacInitValue4=0  parDacReset4=on  parDiChannels=[1 2 3 4 5 6 7 8]  parDoChannels=[9 10 11 12 13 14 15 16]  parDioFirstControl=[2 3 4 5 6 7 8 9]  parDioSecondControl=0  parDioChannel1=In  parExtra1=I  parExtra2=I  parExtra3=I  parDioChannel2=Out  parDioChannel3=Out  parDioChannel4=Out  parDioChannel5=Out  parDioChannel6=Out  parDioChannel7=Out  parDioChannel8=Out  parDioChannel9=Out  parDoInitValues=[0 0 0 0]  parDoResets=[1 1 1 1]  parDoInitValue1=0  parDoReset1=on  parDoInitValue2=0  parDoReset2=on  parDoInitValue3=0  parDoReset3=on  parDoInitValue4=0  parDoReset4=on  parDoInitValue5=0  parDoReset5=on  parDoInitValue6=0  parDoReset6=on  parDoInitValue7=0  parDoReset7=on  parDoInitValue8=0  parDoReset8=on  parDoInitValue9=0  parDoReset9=on  parDoInitValue10=0  parDoReset10=on  parDoInitValue11=0  parDoReset11=on  parDoInitValue12=0  parDoReset12=on  parDoInitValue13=0  parDoReset13=on  parDoInitValue14=0  parDoReset14=on  parDoInitValue15=0  parDoReset15=on  parDoInitValue16=0  parDoReset16=on
      settings: SourceProductName=Simulink Real-Time: Speedgoat I/O Blockset
  TCP Server : slrealtimeiplib/TCP Server  Priority=-1  useHostTargetConn=off  serverAddress=192.168.10.1  serverPort=8001
  Server Status : Outport
  wires:
  Enable Server/1 -> TCP Server/1
  TCP Server/1 -> Server Status/1
